simulink model "thevenin_theorem_v2"  (R2015a)
settings: Solver=ode15s  StartTime=0.0  StopTime=1
libraries: fl_lib x8, nesl_utility x5, elec_lib x2
settings Model: Creator=Asif  LastModifiedBy=Asif
settings DebuggingCC: StateNameClashWarn=warning

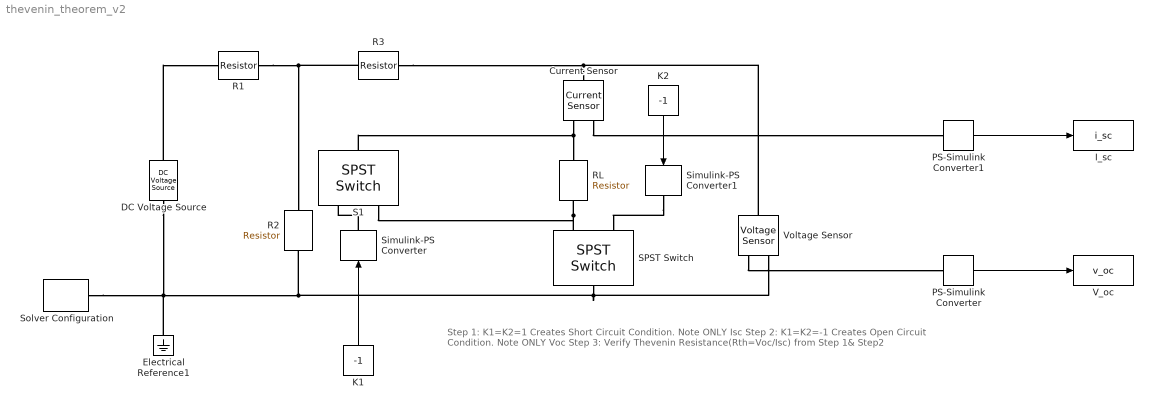
== system thevenin_theorem_v2 ==
  note: Step 1: K1=K2=1 Creates Short Circuit Condition. Note ONLY Isc
      |
      | Step 2: K1=K2=-1 Creates Open Circuit Condition. Note ONLY Voc
      |
      | Step 3: Verify Thevenin Resistance(Rth=Voc/Isc) from Step 1& Step2
  Current Sensor : fl_lib/Electrical/Electrical Sensors/Current Sensor
  DC Voltage Source : fl_lib/Electrical/Electrical Sources/DC Voltage Source  v0=10 V
  Electrical Reference1 : fl_lib/Electrical/Electrical Elements/Electrical Reference
  I_sc : ToWorkspace  VariableName=i_sc  SaveFormat=Timeseries  SampleTime=-1
  K1 : Constant  Value=-1
  K2 : Constant  Value=-1
  PS-Simulink Converter : nesl_utility/PS-Simulink Converter  PhysicalDomain=network_engine_domain  SubClassName=ps_output  LeftPortType=input  RightPortType=output  PseudoPeriodic=off  Frequencies=[]  Unit=1  AffineConversion=off
  PS-Simulink Converter1 : nesl_utility/PS-Simulink Converter  PhysicalDomain=network_engine_domain  SubClassName=ps_output  LeftPortType=input  RightPortType=output  PseudoPeriodic=off  Frequencies=[]  Unit=1  AffineConversion=off
  R1 : fl_lib/Electrical/Electrical Elements/Resistor  R=10 kOhm  i_specify=off  i_priority=High  i=0 A  v_specify=off  v_priority=High  v=0 V
  R2 : fl_lib/Electrical/Electrical Elements/Resistor  R=10 kOhm  i_specify=off  i_priority=High  i=0 A  v_specify=off  v_priority=High  v=0 V
  R3 : fl_lib/Electrical/Electrical Elements/Resistor  R=5 kOhm  i_specify=off  i_priority=High  i=0 A  v_specify=off  v_priority=High  v=0 V
  RL : fl_lib/Electrical/Electrical Elements/Resistor  R=22 kOhm  i_specify=off  i_priority=High  i=0 A  v_specify=off  v_priority=High  v=0 V
  S1 : elec_lib/Passive Devices/Switches/SPST Switch  R_closed=0.01 Ohm  G_open=1e-6 S  Threshold=0 V  Width=0 V  model_dynamics=0  t_on=0.001 s  t_off=0.001 s  initial_vT=0 V
  SPST Switch : elec_lib/Passive Devices/Switches/SPST Switch  R_closed=0.01 Ohm  G_open=1e-6 S  Threshold=0 V  Width=0 V  model_dynamics=0  t_on=0.001 s  t_off=0.001 s  initial_vT=0 V
  Simulink-PS Converter : nesl_utility/Simulink-PS Converter  PhysicalDomain=network_engine_domain  SubClassName=ps_input  LeftPortType=input  RightPortType=output  PseudoPeriodic=off  Frequencies=[]  NoiseDistribution=none  NoiseParameters=[]  Unit=1  AffineConversion=off  InputFiltering=off  SimscapeFilterOrder=1  InputFilterTimeConstant=0.001  UdotUserProvided=1
  Simulink-PS Converter1 : nesl_utility/Simulink-PS Converter  PhysicalDomain=network_engine_domain  SubClassName=ps_input  LeftPortType=input  RightPortType=output  PseudoPeriodic=off  Frequencies=[]  NoiseDistribution=none  NoiseParameters=[]  Unit=1  AffineConversion=off  InputFiltering=off  SimscapeFilterOrder=1  InputFilterTimeConstant=0.001  UdotUserProvided=1
  Solver Configuration : nesl_utility/Solver Configuration  PhysicalDomain=network_engine_domain  SubClassName=solver  LeftPortType=input  RightPortType=generic  Accelerate=off  Tones=[]  Harmonics=[]  SimulateNoise=off  Profile=off  UseLocalSampling=off  EnableSwitchedLinearOptims=on  FrequencyDomain=off  UseCCode=off  RelTol=0.001  AbsTol=1e-06  MinStep=1e-09  ToWorkspace=off  RevertToSquareIcSolve=off  NumHomotopyIterations=100  DoDC=on  ResidualTolerance=1e-09  UseLocalSolver=off  LocalSolverChoice=NE_BACKWARD_EULER_ADVANCER  LocalSolverSampleTime=1e-6  DoFixedCost=off  MaxNonlinIter=3  MaxModeIter=2  LinearAlgebra=Sparse  DelaysMemoryBudget=1024  AutomaticFiltering=on  FilteringTimeConstant=0.001
  V_oc : ToWorkspace  VariableName=v_oc  SaveFormat=Timeseries  SampleTime=-1
  Voltage Sensor : fl_lib/Electrical/Electrical Sensors/Voltage Sensor
  wires:
  PS-Simulink Converter/1 -> V_oc/1
  PS-Simulink Converter1/1 -> I_sc/1
  K1/1 -> Simulink-PS Converter/1
  K2/1 -> Simulink-PS Converter1/1
  connections:
  R1/RConn1 -- R2/LConn1 -- R3/RConn1
  Electrical Reference1/LConn1 -- SPST Switch/RConn1 -- Voltage Sensor/RConn2 -- R2/RConn1 -- DC Voltage Source/RConn1 -- Solver Configuration/RConn1
  Voltage Sensor/RConn1 -- PS-Simulink Converter/LConn1
  DC Voltage Source/LConn1 -- R1/LConn1
  R3/LConn1 -- Voltage Sensor/LConn1 -- Current Sensor/LConn1
  Current Sensor/RConn2 -- RL/LConn1 -- S1/RConn1
  Current Sensor/RConn1 -- PS-Simulink Converter1/LConn1
  S1/LConn2 -- SPST Switch/LConn2 -- RL/RConn1
  Simulink-PS Converter/RConn1 -- S1/LConn1
  Simulink-PS Converter1/RConn1 -- SPST Switch/LConn1
